simulink model "r_1f_2bx_8a_1k_r365"  (R2012b)
(part 2 of 67)

  [vacc_ld_time] -> vacc0/3(load_time)
  [vacc_rst] -> vacc0/1(rst)
  vacc_ld_status0/1(sim_reg_out) -> Terminator4/1
  vacc_tvg1/1(sync_out) -> vacc1/5(sync_in)
  vacc_tvg1/2(data_out) -> vacc1/6(data_in)
  vacc_tvg1/3(valid_out) -> vacc1/7(we)
  [acc_len] -> vacc1/4(acc_len)
  xeng1/4(mcnt_out) -> delay1/1
  [vacc_ld_arm] -> vacc1/2(arm)
  [vacc_ld_time] -> vacc1/3(load_time)
  [vacc_rst] -> vacc1/1(rst)
  vacc_ld_status1/1(sim_reg_out) -> Terminator3/1
  delay5/1 -> vacc0/8(pcnt_in)
  delay1/1 -> vacc1/8(pcnt_in)
  vacc0/10(error_out) -> [vacc_err0]
  [new_acc0] -> vacc_monitor/2(new_acc)
  [vacc_err0] -> vacc_monitor/3(error)
  pkt_reord0/2(data_out) -> Delay21/1(d), Subsystem14/2(dout)
  [board_id] -> pkt_reord0/7(board_id)
  pkt_reord0/8(xeng_id) -> [id0]
  pkt_reord1/1(sync_out) -> [x_sync1], Delay49/1(d), Subsystem1/1(sync), miss_cnt1/2(sync)
  pkt_reord1/2(data_out) -> Delay50/1(d), Subsystem1/2(dout)
  pkt_reord1/3(valid_out) -> miss_cnt1/3(valid), Delay51/1(d), Subsystem1/3(valid)
  pkt_reord1/4(mcnt_out) -> Delay52/1(d), Subsystem1/4(mcnt)
  pkt_reord0/6(flag_out) -> Subsystem14/5(flag)
  [board_id] -> pkt_reord1/7(board_id)
  pkt_reord1/8(xeng_id) -> [id1]
  pkt_reord1/5(rcvd) -> miss_cnt1/4(rcvd), Subsystem1/6(rcvd)
  [new_acc1] -> Logical2/1
  [new_acc0] -> Logical2/2
  Logical2/1 -> Delay118/1(d)
  Delay27/1(q) -> negedge_delay2/1
  Inverter/1 -> Delay27/1(d)
  [gbe_up] -> Inverter/1
  Delay96/1(q) -> negedge_delay3/1
  Logical4/1 -> Delay96/1(d)
  [xeng_err0] -> Logical4/1
  [xeng_err1] -> Logical4/2
  Delay97/1(q) -> negedge_delay4/1
  Logical5/1 -> Delay97/1(d)
  [vacc_err0] -> Logical5/1
  [vacc_err1] -> Logical5/2
  miss_cnt0/4(err_now) -> [xeng_err0]
  miss_cnt1/4(err_now) -> [xeng_err1]
  Constant10/1 -> Delay147/1(d)
  Constant11/1 -> Delay148/1(d)
  Constant16/1 -> miss_cnt0/5(err), [pkt_reord_err0]
  Constant17/1 -> miss_cnt1/5(err), [pkt_reord_err1]
  Subsystem1/1(data) -> Delay1/1(d)
  Subsystem1/2(we) -> Delay3/1(d)
  Subsystem1/3(trig) -> Delay4/1(d)
  Subsystem1/4(stop) -> Delay5/1(d)
  pkt_reord1/6(flag_out) -> Subsystem1/5(flag)
  vacc0/2(data_out) -> delay4/1
  vacc0/4(valid_out) -> delay2/1
  vacc0/6(rb_done) -> delay6/1
  vacc0/5(pkt_rdy) -> [vacc_pkt_rdy0]
  [vacc_ld_stat0] -> vacc_ld_status0/1(reg_out)
  vacc0/8(ld_status) -> [vacc_ld_stat0]
  [id0] -> pack_out0/6(xeng_id)
  [cnt_rst] -> vacc_monitor1/1(cnt_rst)
  [vacc_err1] -> vacc_monitor1/3(error)
  [new_acc1] -> vacc_monitor1/2(new_acc)
  vacc1/1(new_acc) -> [new_acc1]
  vacc1/2(data_out) -> delay16/1
  vacc1/4(valid_out) -> delay17/1
  vacc1/5(pkt_rdy) -> [vacc_pkt_rdy1]
  vacc1/6(rb_done) -> delay19/1
  vacc1/7(timestamp) -> delay20/1
  [id1] -> pack_out1/6(xeng_id)
  vacc1/8(ld_status) -> [vacc_ld_stat1]
  vacc1/10(error_out) -> [vacc_err1]
  [vacc_ld_stat1] -> vacc_ld_status1/1(reg_out)
  pack_out1/5(fetch) -> vacc1/9(re)
  [vacc_err0] -> snap_xeng1/4(stop)
  pack_out0/3(eof) -> Delay15/1(d)
  Constant2/1 -> [gbe_rxack]
  pack_out_err0/1(sim_reg_out) -> Terminator6/1
  pack_out_cnt0/1(sim_reg_out) -> Terminator5/1
  [cnt_rst] -> vacc_monitor2/1(cnt_rst)
  vacc_monitor2/1(pkt_cnt) -> pack_out_cnt0/1(reg_out)
  vacc_monitor2/2(error_cnt) -> pack_out_err0/1(reg_out)
  pack_out_err1/1(sim_reg_out) -> Terminator21/1
  pack_out_cnt1/1(sim_reg_out) -> Terminator12/1
  [cnt_rst] -> vacc_monitor3/1(cnt_rst)
  vacc_monitor3/1(pkt_cnt) -> pack_out_cnt1/1(reg_out)
  vacc_monitor3/2(error_cnt) -> pack_out_err1/1(reg_out)
  pack_out1/3(eof) -> Delay11/1(d)
  pack_out0/5(fetch) -> vacc0/9(re)
  delay4/1 -> snap_xeng1/1(din), pack_out0/1(data_in)
  delay2/1 -> snap_xeng1/2(we), pack_out0/2(valid_in)
  delay6/1 -> pack_out0/4(rb_done), snap_xeng1/3(trig)
  delay7/1 -> pack_out0/5(timestamp)
  delay16/1 -> pack_out1/1(data_in)
  delay17/1 -> pack_out1/2(valid_in)
  delay19/1 -> pack_out1/4(rb_done)
  delay20/1 -> pack_out1/5(timestamp)
  pack_out0/1(data_out) -> Delay23/1(d)
  pack_out0/2(valid_out) -> Logical/2
  Delay23/1(q) -> [vacc_dout0]
  Logical/1 -> [vacc_valid0]
  Delay15/1(q) -> [vacc_eof0]
  Delay14/1(q) -> [vacc_dout1]
  Delay11/1(q) -> [vacc_eof1]
  pack_out1/1(data_out) -> Delay14/1(d)
  [vacc_eof1] -> vacc_monitor3/2(eof)
  Delay33/1(q) -> [pack_err1]
  pack_out1/4(err) -> Delay33/1(d)
  [pack_err1] -> vacc_monitor3/3(error)
  Delay34/1(q) -> [pack_err0]
  pack_out0/4(err) -> Delay34/1(d)
  [vacc_eof0] -> vacc_monitor2/2(eof)
  [pack_err0] -> vacc_monitor2/3(error)
  delay8/1 -> gbe0/1
  delay9/1 -> gbe0/2
  delay10/1 -> gbe0/3
  delay11/1 -> gbe0/4
  delay12/1 -> gbe0/5
  delay13/1 -> gbe0/6
  delay14/1 -> gbe0/7
  delay15/1 -> gbe0/8
  [tx_pkt0] -> pack_out0/3(pkt_rdy)
  [tx_pkt1] -> pack_out1/3(pkt_rdy)
  Slice6/1 -> Delay44/1(d)
  Delay44/1(q) -> [flasher_en]
  Constant1/1 -> front_panel/5(led1_red)
  negedge_delay3/1 -> front_panel/6(led2_red)
  negedge_delay4/1 -> front_panel/7(led3_red)
  Constant15/1 -> front_panel/8(led4_green)
  Inverter1/1 -> led0_10gbe_fault/1
  Inverter2/1 -> led1_xaui_sync/1
  Inverter3/1 -> led2_x_sync/1
  Inverter4/1 -> led3_new_acc/1
  [flasher_en] -> front_panel/1(flasher_en)
  [new_acc0] -> front_panel/2(sync)
  [x_sync0] -> front_panel/3(step)
  pkt_reord_cnt1/1(sim_reg_out) -> Terminator22/1
  pkt_reord_err1/1(sim_reg_out) -> Terminator23/1
  last_missing_ant1/1(sim_reg_out) -> Terminator2/1
  xstatus0/1(sim_reg_out) -> Terminator24/1
  Subsystem6/1(status) -> xstatus0/1(reg_out)
  [clr_status] -> Subsystem6/1(clr)
  negedge_delay2/1 -> front_panel/4(led0_red), Inverter1/1
  negedge_delay/1 -> front_panel/10(led6_green), Inverter3/1
  negedge_delay1/1 -> front_panel/9(led5_green), Inverter4/1
  Constant5/1 -> front_panel/11(led7_green)
  Slice10/1 -> Delay13/1(d)
  Delay13/1(q) -> [clr_status]
  Inverter5/1 -> Subsystem6/2(gbe_down)
  [gbe_up] -> Inverter5/1
  [xeng_err0] -> Subsystem6/3(xeng_err)
  [vacc_err0] -> Subsystem6/4(vacc_err)
  [rx_bad_pkt] -> Subsystem6/5(rx_bad_pkt)
  [gbe_rx_bad] -> Subsystem6/6(rx_bad_frame)
  [gbe_tx_over] -> Subsystem6/7(tx_over)
  [pkt_reord_err0] -> Subsystem6/8(pkt_reord_err)
  [pack_err0] -> Subsystem6/9(pack_err)
  xstatus1/1(sim_reg_out) -> Terminator27/1
  Subsystem7/1(status) -> xstatus1/1(reg_out)
  [clr_status] -> Subsystem7/1(clr)
  Inverter6/1 -> Subsystem7/2(gbe_down)
  [gbe_up] -> Inverter6/1
  [xeng_err1] -> Subsystem7/3(xeng_err)
  [vacc_err1] -> Subsystem7/4(vacc_err)
  [rx_bad_pkt] -> Subsystem7/5(rx_bad_pkt)
  [gbe_rx_bad] -> Subsystem7/6(rx_bad_frame)
  [gbe_tx_over] -> Subsystem7/7(tx_over)
  [pkt_reord_err1] -> Subsystem7/8(pkt_reord_err)
  [pack_err1] -> Subsystem7/9(pack_err)
  Delay1/1(q) -> snap_descramble1/1(din)
  Delay3/1(q) -> snap_descramble1/2(we)
  Delay4/1(q) -> snap_descramble1/3(trig)
  Delay5/1(q) -> snap_descramble1/4(stop)
  Delay42/1(q) -> snap_descramble0/2(we)
  Delay43/1(q) -> snap_descramble0/3(trig)
  Subsystem3/1(data_out) -> snap_gbe_tx0/1(din)
  Subsystem3/2(we_out) -> snap_gbe_tx0/2(we)
  Subsystem3/3(trig_out) -> snap_gbe_tx0/3(trig)
  prep_snap_rx0/1(data_out) -> snap_rx0/1(din)
  prep_snap_rx0/2(we_out) -> snap_rx0/2(we)
  prep_snap_rx0/3(trig_out) -> snap_rx0/3(trig)
  Subsystem4/1(data_out) -> snap_gbe_rx0/1(din)
  Subsystem4/2(we_out) -> snap_gbe_rx0/2(we)
  Subsystem4/3(trig_out) -> snap_gbe_rx0/3(trig)
  Constant4/1 -> bf0/4(badi)
  Constant7/1 -> bf0/6(misci)
  Slice11/1 -> [bf0_pol0]
  Slice12/1 -> [bf0_pol1]
  bf0/5(misco) -> Terminator/1
  Slice15/1 -> [bf0_eno0]
  Slice16/1 -> [bf0_eno1]
  Delay32/1(q) -> bf0/1(synci)
  Delay45/1(q) -> bf0/2(di)
  Delay46/1(q) -> bf0/3(deni)
  Delay47/1(q) -> round_pcnt0/1(In1)
  Delay57/1(q) -> round_pcnt1/1(In1)
  Delay16/1 -> [gbe_txvld]
  Concat/1 -> gbe_mux_bus/2(di)
  gbe_mux_bus/3(valido) -> Delay16/1
  gbe_mux_bus/4(eofo) -> Delay104/1
  gbe_mux_bus/5(start) -> Delay106/1
  [bf0s_en0] -> Concat1/1
  [bf0s_en1] -> Concat1/2
  [bf1s_en0] -> Concat1/3
  [bf1s_en1] -> Concat1/4
  [vacc_valid0] -> Concat1/5
  [vacc_valid1] -> Concat1/6
  [bf0s_eof0] -> Concat3/1
  [bf0s_eof1] -> Concat3/2
  [bf1s_eof0] -> Concat3/3
  [bf1s_eof1] -> Concat3/4
  [vacc_eof0] -> Concat3/5
  [vacc_eof1] -> Concat3/6
  Concat1/1 -> gbe_mux_bus/3(validi)
  Concat3/1 -> gbe_mux_bus/4(eofi)
  Concat5/1 -> gbe_mux_bus/5(drdy)
  [bf0s_pkt_ready0] -> Concat5/1
  [bf0s_pkt_ready1] -> Concat5/2
  [bf1s_pkt_ready0] -> Concat5/3
  [bf1s_pkt_ready1] -> Concat5/4
  [vacc_pkt_rdy0] -> Concat5/5
  [vacc_pkt_rdy1] -> Concat5/6
  bus_expand/5(out2) -> [tx_pkt0]
  bus_expand/6(lsb_out1) -> [tx_pkt1]
  bus_expand/1(msb_out6) -> [bf0_tx_pkt0]
  bus_expand/2(out5) -> [bf0_tx_pkt1]
  bus_expand/3(out4) -> [bf1_tx_pkt0]
  bus_expand/4(out3) -> [bf1_tx_pkt1]
  Register/1 -> [bf0s_d0]
  Delay68/1 -> [bf0s_eof0]
  Delay71/1 -> [bf0s_pkt_ready0]
  [gbe_out_rst] -> gbe_mux_bus/1(rst)
  Constant22/1 -> [beng_data_id]
  [bf0s_d0] -> Concat/1
  [bf0s_d1] -> Concat/2
  [bf1s_d0] -> Concat/3
  [bf1s_d1] -> Concat/4
  [vacc_dout0] -> Concat/5
  [vacc_dout1] -> Concat/6
  gbe_mux_bus/2(do) -> Delay114/1
  Delay114/1 -> [gbe_txd]
  Delay104/1 -> [gbe_txeof]
  Delay106/1 -> bus_expand/1(bus_in)
  round_pcnt0/1(Out1) -> bf0/5(timei)
  [bf0_synco] -> speadify0/2(synci)
  [bf0_tx_pkt0] -> speadify0/6(start)
  Constant13/1 -> bf0_cfg0/1
  [bf0_pol0] -> speadify0/3(di)
  [bf0_eno0] -> speadify0/4(eni)
  [bf0_timeo] -> speadify0/5(timei)
  Constant/1 -> bf0_dest/2(data_in)
  Constant23/1 -> bf0_dest/3(we)
  Constant20/1 -> bf1_dest/2(data_in)
  Constant21/1 -> bf1_dest/3(we)
  gbe_mux_bus/1(input) -> Slice22/1, Slice23/1, Slice24/1
  err_clear_sim1/1 -> gbe_out_port/1
  gbe_out_port/1 -> Delay9/1(d)
  Delay9/1(q) -> [gbe_out_txport]
  err_clear_sim5/1 -> gbe_out_ip/1
  gbe_out_ip/1 -> Delay10/1(d)
  Delay10/1(q) -> [gbe_out_ip_addr]
  Slice23/1 -> bf0_dest/1(addr)
  Slice24/1 -> bf1_dest/1(addr)
  bf1_dest/1(data_out) -> Slice25/1, Slice26/1
  Mux1/1 -> [gbe_txport]
  Slice21/1 -> Mux1/2
  Slice22/1 -> Mux1/1, Mux2/1
  [gbe_out_txport] -> Mux1/4
  Slice/1 -> Mux2/2
  [gbe_out_ip_addr] -> Mux2/4
  Mux2/1 -> [gbe_txip]
  speadify0/1(do) -> Register/1
  speadify0/2(eno) -> Delay93/1, Register/2
  speadify0/3(eofo) -> Delay68/1
  speadify0/4(pkt_ready) -> Delay71/1
  bf0_cfg0/1 -> comp_index0/1, n_comps0/1, rst0/1, beam_id0/1
  [gbe_out_enable] -> Logical/1
  pack_out1/2(valid_out) -> Logical1/2
  [gbe_out_enable] -> Logical1/1
  Logical1/1 -> [vacc_valid1]
  Slice25/1 -> Mux2/3
  Slice26/1 -> Mux1/3
  bf0_dest/1(data_out) -> Slice21/1, Slice/1
  bf0/4(timeo) -> [bf0_timeo]
  bf0/1(synco) -> [bf0_synco]
  bf0/3(deno) -> Slice16/1, Slice15/1
  bf0/2(do) -> Slice12/1, Slice11/1
  bf1/5(misco) -> Terminator28/1
  bf1/4(timeo) -> [bf1_timeo]
  bf1/1(synco) -> [bf1_synco]
  bf1/3(deno) -> Slice20/1, Slice19/1
  bf1/2(do) -> Slice18/1, Slice17/1
  Slice17/1 -> [bf1_pol0]
  Slice18/1 -> [bf1_pol1]
  Slice19/1 -> [bf1_eno0]
  Slice20/1 -> [bf1_eno1]
  Delay48/1(q) -> bf1/1(synci)
  Delay54/1(q) -> bf1/2(di)
  Delay55/1(q) -> bf1/3(deni)
  Constant8/1 -> bf1/4(badi)
  round_pcnt1/1(Out1) -> bf1/5(timei)
  Constant9/1 -> bf1/6(misci)
  Delay93/1 -> [bf0s_en0]
  comp_index0/1 -> speadify0/10(partition)
  [beng_time_id] -> speadify0/7(time_id)
  n_comps0/1 -> speadify0/9(n_partitions)
  [beng_data_id] -> Concat2/1
  beam_id0/1 -> Concat2/2
  Concat2/1 -> speadify0/8(data_id)
  Constant24/1 -> [beng_time_id]
  Constant25/1 -> Concat7/1
  Concat7/1 -> bf0_status0/1
  bf0_status0/1 -> Terminator29/1
  speadify0/5(of) -> Register4/1, Register4/3
  [clr_status] -> Register4/2
  Register4/1 -> Concat7/2
  Constant28/1 -> Concat11/1
  Concat11/1 -> bf1_status1/1
  bf1_status1/1 -> Terminator33/1
  Register7/1 -> Concat11/2
  [bf0_synco] -> snap_bf0_pol0/3(trig)
  [bf0_eno0] -> snap_bf0_pol0/2(we)
  [bf0_pol0] -> snap_bf0_pol0/1(din)
  [bf0_synco] -> snap_bf0_pol1/3(trig)
  [bf0_eno1] -> snap_bf0_pol1/2(we)
  [bf0_pol1] -> snap_bf0_pol1/1(din)
  [bf1_synco] -> snap_bf1_pol0/3(trig)
  [bf1_eno0] -> snap_bf1_pol0/2(we)
  [bf1_pol0] -> snap_bf1_pol0/1(din)
  [bf1_synco] -> snap_bf1_pol1/3(trig)
  [bf1_eno1] -> snap_bf1_pol1/2(we)
  [bf1_pol1] -> snap_bf1_pol1/1(din)
  [bf0_synco] -> speadify1/2(synci)
  [bf0_tx_pkt1] -> speadify1/6(start)
  Constant14/1 -> bf0_cfg1/1
  [bf0_pol1] -> speadify1/3(di)
  [bf0_eno1] -> speadify1/4(eni)
  [bf0_timeo] -> speadify1/5(timei)
  bf0_cfg1/1 -> beam_id2/1, rst1/1, n_comps2/1, comp_index2/1
  comp_index2/1 -> speadify1/10(partition)
  [beng_time_id] -> speadify1/7(time_id)
  n_comps2/1 -> speadify1/9(n_partitions)
  [beng_data_id] -> Concat4/1
  beam_id2/1 -> Concat4/2
  Concat4/1 -> speadify1/8(data_id)
  rst1/1 -> speadify1/1(rst)
  speadify1/1(do) -> Register1/1
  speadify1/2(eno) -> Register1/2, Delay101/1
  speadify1/3(eofo) -> Delay77/1
  speadify1/4(pkt_ready) -> Delay98/1
  Register1/1 -> [bf0s_d1]
  Delay101/1 -> [bf0s_en1]
  Delay77/1 -> [bf0s_eof1]
  Delay98/1 -> [bf0s_pkt_ready1]
  Constant26/1 -> Concat9/1
  Concat9/1 -> bf0_status1/1
  bf0_status1/1 -> Terminator31/1
  speadify1/5(of) -> Register5/1, Register5/3
  [clr_status] -> Register5/2
  Register5/1 -> Concat9/2
  [bf1_synco] -> speadify2/2(synci)
  [bf1_tx_pkt0] -> speadify2/6(start)
  Constant18/1 -> bf1_cfg0/1
  [bf1_pol0] -> speadify2/3(di)
  [bf1_eno0] -> speadify2/4(eni)
  [bf1_timeo] -> speadify2/5(timei)
  bf1_cfg0/1 -> comp_index1/1, n_comps1/1, rst2/1, beam_id1/1
  comp_index1/1 -> speadify2/10(partition)
  [beng_time_id] -> speadify2/7(time_id)
  n_comps1/1 -> speadify2/9(n_partitions)
  [beng_data_id] -> Concat6/1
  beam_id1/1 -> Concat6/2
  Concat6/1 -> speadify2/8(data_id)
  rst2/1 -> speadify2/1(rst)
  speadify2/1(do) -> Register2/1
  speadify2/2(eno) -> Delay69/1, Register2/2
  speadify2/3(eofo) -> Delay99/1
  speadify2/4(pkt_ready) -> Delay102/1
  Register2/1 -> [bf1s_d0]
  Delay69/1 -> [bf1s_en0]
  Delay99/1 -> [bf1s_eof0]
  Delay102/1 -> [bf1s_pkt_ready0]
  speadify2/5(of) -> Register6/1, Register6/3
  [clr_status] -> Register6/2
  Constant27/1 -> Concat10/1
  Concat10/1 -> bf1_status0/1
  bf1_status0/1 -> Terminator32/1
  Register6/1 -> Concat10/2
  [bf1_synco] -> speadify3/2(synci)
  [bf1_tx_pkt1] -> speadify3/6(start)
  Constant19/1 -> bf1_cfg1/1
  [bf1_eno1] -> speadify3/4(eni)
  [bf1_timeo] -> speadify3/5(timei)
  bf1_cfg1/1 -> beam_id3/1, rst3/1, n_comps3/1, comp_index3/1
  comp_index3/1 -> speadify3/10(partition)
  [beng_time_id] -> speadify3/7(time_id)
  n_comps3/1 -> speadify3/9(n_partitions)
  [beng_data_id] -> Concat8/1
  beam_id3/1 -> Concat8/2
  Concat8/1 -> speadify3/8(data_id)
  rst3/1 -> speadify3/1(rst)
  speadify3/1(do) -> Register3/1
  speadify3/2(eno) -> Register3/2, Delay103/1
  speadify3/3(eofo) -> Delay105/1
  speadify3/4(pkt_ready) -> Delay31/1
  speadify3/5(of) -> Register7/1, Register7/3
  [clr_status] -> Register7/2
  Register3/1 -> [bf1s_d1]
  Delay103/1 -> [bf1s_en1]
  Delay105/1 -> [bf1s_eof1]
  Delay31/1 -> [bf1s_pkt_ready1]
  [bf1_pol1] -> speadify3/3(di)
  rst0/1 -> speadify0/1(rst)
